simulink model "AudioPlayer"  (R2017a)
settings: Solver=VariableStepAuto  StartTime=0.0  StopTime=inf  RelTol=1e-3
settings Model: Creator=teobaiguera  LastModifiedBy=teobaiguera

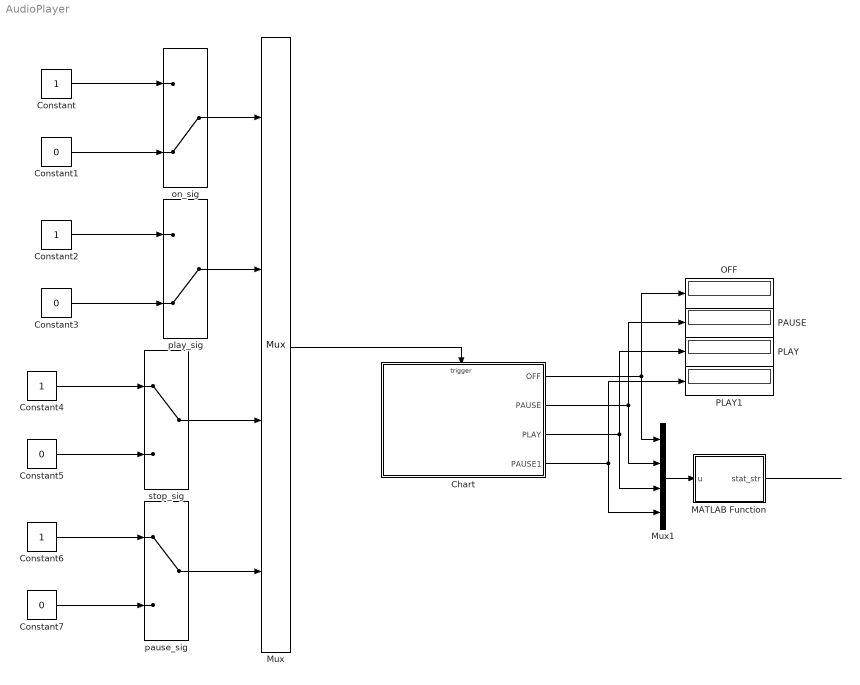
== system AudioPlayer ==
  Chart : Stateflow chart  TreatAsAtomicUnit=on
  Constant{,2,4,6} (4 alike) : Constant
  Constant{1,3,5,7} (4 alike) : Constant  Value=0
  MATLAB Function : MATLAB Function  TreatAsAtomicUnit=on
  Mux : Mux
  Mux1 : Mux
  OFF : Display
  PAUSE : Display
  PLAY : Display
  PLAY1 : Display
  on_sig : ManualSwitch  CurrentSetting=0
  pause_sig : ManualSwitch
  play_sig : ManualSwitch  CurrentSetting=0
  stop_sig : ManualSwitch
  wires:
  Constant/1 -> on_sig/1
  Constant1/1 -> on_sig/2
  Chart/1(" OFF") -> OFF/1, Mux1/1
  Chart/2(" PAUSE") -> PAUSE/1, Mux1/2
  Chart/3(" PLAY") -> PLAY/1, Mux1/3
  Constant2/1 -> play_sig/1
  Constant3/1 -> play_sig/2
  play_sig/1 -> Mux/2
  on_sig/1 -> Mux/1
  Mux/1 -> Chart/Trigger
  Constant4/1 -> stop_sig/1
  Constant5/1 -> stop_sig/2
  stop_sig/1 -> Mux/3
  pause_sig/1 -> Mux/4
  Constant7/1 -> pause_sig/2
  Constant6/1 -> pause_sig/1
  Chart/4(PAUSE1) -> PLAY1/1, Mux1/4
  Mux1/1 -> MATLAB Function/1(u)
  MATLAB Function/1(stat_str) -> ?

== matlab function AudioPlayer/MATLAB Function ==
  data: u input; stat_str output
function stat_str = current_state(u)

stat_str = strings(1)

    if y[1]==1
    stat_str = 'OFF'
    else if y[2] ==1
        stat_str = 'STOP'
    else if y[3] ==1 
        stat_str = 'PLAY'
    else if y[4] ==1
        stat_str = 'PAUSE'

 end
return

== stateflow chart AudioPlayer/Chart ==
  state OFF
  state STOP
  state PLAY
  state PAUSE
  PLAY -> PAUSE [order 3] : pause_sig
  STOP -> PLAY [order 2] : play_sig
  (default) -> OFF
  OFF -> STOP : on_sig
  PLAY -> OFF [order 1] : on_sig
  STOP -> OFF [order 1] : on_sig
  PLAY -> STOP [order 2] : stop_sig
  PAUSE -> PLAY : play_sig
  data: OFF output boolean; PAUSE output boolean; PLAY output boolean; PAUSE1 output boolean
  events: event local FUNCTION_CALL_EVENT; on_sig input EITHER_EDGE_EVENT; play_sig input EITHER_EDGE_EVENT; stop_sig input EITHER_EDGE_EVENT; pause_sig input EITHER_EDGE_EVENT
